simulink model "lateral_pendulum_planar_moving_vehicle_sim"  (R2024b)
settings: Solver=ode4  StartTime=0.0  StopTime=time_arr(end)  FixedStep=ts  RelTol=1e-3
values from neighbouring files (symbols this model uses):
  c = 0.0    (= 0)    [curvature_optimal_sequence_example_vel_lim.m]    (also in optimal_sequence_example.m = 0.1; time_optimal_sequence_example_vel_lim.m; yas_marina_optimal_sequence.m = 0.1)
  lw = 2.0    (= 2)    [curvature_optimal_sequence_example_vel_lim.m]    (also in no_vel_curvature_optimal_sequence.m = 2.971; optimal_sequence_example.m; time_optimal_sequence_example_vel_lim.m; yas_marina_optimal_sequence.m)
  ts = 0.01    [curvature_optimal_sequence_example_vel_lim.m]    (also in time_optimal_sequence_example_vel_lim.m; yas_marina_optimal_sequence.m)
  v0 = 10.0    (= 10)    [curvature_optimal_sequence_example_vel_lim.m]    (also in no_vel_curvature_optimal_sequence.m = 1; optimal_sequence_example.m = 1; time_optimal_sequence_example_vel_lim.m; yas_marina_optimal_sequence.m)
  x_y_yaw_curv_s_lx_ly_rx_ry_dl_dr = spline_x_y_yaw_curv_s_lx_ly_rx_ry_dl_dr    [curvature_optimal_sequence_example_vel_lim.m]    (also in no_vel_curvature_optimal_sequence.m)
settings Model: Creator=Bugra  LastModifiedBy=Bugra

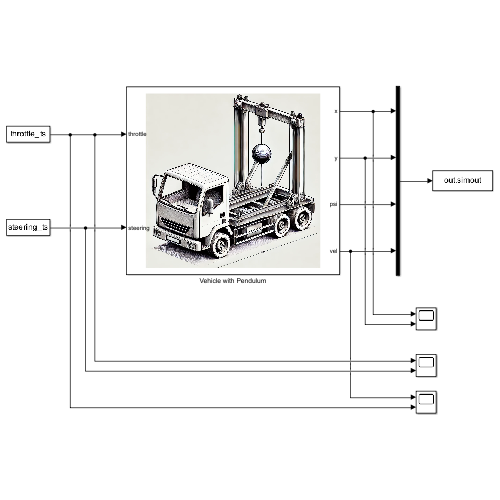
[thumbnail: Simulink's stored preview of the top-level diagram]
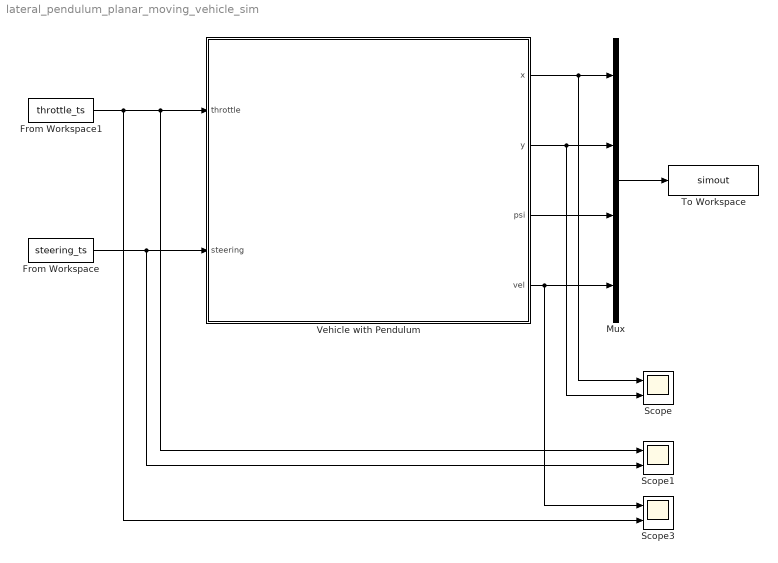
== system lateral_pendulum_planar_moving_vehicle_sim ==
  From Workspace : FromWorkspace  VariableName=steering_ts  SampleTime=ts  Interpolate=off  OutputAfterFinalValue=Holding final value
  From Workspace1 : FromWorkspace  VariableName=throttle_ts  SampleTime=ts  Interpolate=off  OutputAfterFinalValue=Holding final value
  Mux : Mux
  Scope : Scope  NumInputPorts=2
  Scope1 : Scope  NumInputPorts=2
  Scope3 : Scope  NumInputPorts=2
  To Workspace : ToWorkspace  VariableName=simout  SampleTime=-1
  Vehicle with Pendulum : Subsystem
      mask Display: image('pendulum_on_vehicle.png', [10,10,10,10,100,100]);
  wires:
  Vehicle with Pendulum/4(vel) -> Scope3/1, Mux/4
  Vehicle with Pendulum/3(psi) -> Mux/3
  Vehicle with Pendulum/2(y) -> Scope/2, Mux/2
  Vehicle with Pendulum/1(x) -> Scope/1, Mux/1
  Mux/1 -> To Workspace/1
  From Workspace/1 -> Scope1/2, Vehicle with Pendulum/2(steering)
  From Workspace1/1 -> Scope3/2, Scope1/1, Vehicle with Pendulum/1(throttle)

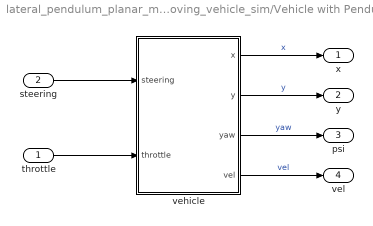
== system lateral_pendulum_planar_moving_vehicle_sim/Vehicle with Pendulum ==
  throttle : Inport
  steering : Inport  Port=2
  vehicle : Subsystem
  x : Outport
  y : Outport  Port=2
  psi : Outport  Port=3
  vel : Outport  Port=4
  wires:
  throttle/1 -> vehicle/2(throttle)
  steering/1 -> vehicle/1(steering)
  vehicle/1(x) -> x/1  "x"
  vehicle/2(y) -> y/1  "y"
  vehicle/3(yaw) -> psi/1  "yaw"
  vehicle/4(vel) -> vel/1  "vel"

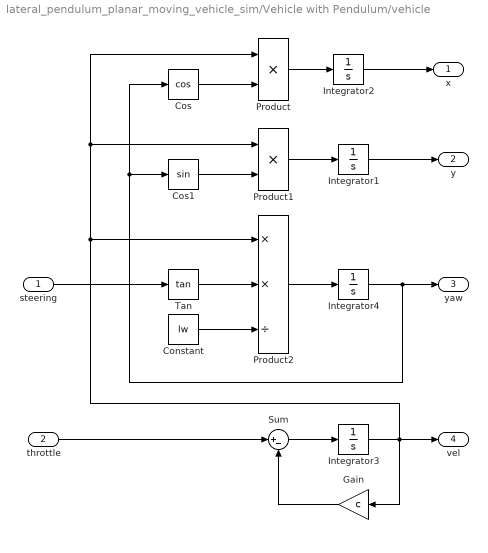
== system lateral_pendulum_planar_moving_vehicle_sim/Vehicle with Pendulum/vehicle ==
  steering : Inport
  throttle : Inport  Port=2
  Constant : Constant  Value=lw
  Cos : Trigonometry  Operator=cos
  Cos1 : Trigonometry
  Gain : Gain  Gain=c
  Integrator1 : Integrator  InitialCondition=x_y_yaw_curv_s_lx_ly_rx_ry_dl_dr(1,2)
  Integrator2 : Integrator  InitialCondition=x_y_yaw_curv_s_lx_ly_rx_ry_dl_dr(1,1)
  Integrator3 : Integrator  InitialCondition=v0
  Integrator4 : Integrator  InitialCondition=x_y_yaw_curv_s_lx_ly_rx_ry_dl_dr(1,3)
  Product : Product
  Product1 : Product
  Product2 : Product  Inputs=**/
  Sum : Sum  Inputs=|+-
  Tan : Trigonometry  Operator=tan
  x : Outport
  y : Outport  Port=2
  yaw : Outport  Port=3
  vel : Outport  Port=4
  wires:
  Product2/1 -> Integrator4/1
  Integrator4/1 -> Cos/1, Cos1/1, yaw/1
  Integrator3/1 -> Product/1, Product1/1, Product2/1, vel/1, Gain/1
  Integrator2/1 -> x/1
  Product/1 -> Integrator2/1
  Cos/1 -> Product/2
  Integrator1/1 -> y/1
  Cos1/1 -> Product1/2
  Product1/1 -> Integrator1/1
  steering/1 -> Tan/1
  Tan/1 -> Product2/2
  Constant/1 -> Product2/3
  Sum/1 -> Integrator3/1
  Gain/1 -> Sum/2
  throttle/1 -> Sum/1
